simulink model "MJAUV_Maneuverability_model_V2"  (R2022b)
settings: Solver=ode4  StartTime=0.0  StopTime=50  FixedStep=0.0001  RelTol=1e-3  EnableMultiTasking=on
libraries: sharedutil x64, matrix_library x35
(part 2 of 5)

== system MJAUV_Maneuverability_model_V2/MJ-AUV Model & PropulsionSystem/Dynamics and Kinematics/6 DOF transformation/E1(e) ==
  note: qo
  note: q1,q2,q3
  e : Inport
  Gain : Gain  Gain=2  SaturateOnIntegerOverflow=on  OutDataTypeStr=Inherit: Same as input  ParamDataTypeStr=Inherit: Same as input
  "Gain " : Gain  Gain=2  SaturateOnIntegerOverflow=on  OutDataTypeStr=Inherit: Same as input  ParamDataTypeStr=Inherit: Same as input
  I (3x3) : Constant  Value=eye(3)
  Matrix Multiply : Product  Multiplication=Matrix(*)
  Product : Product  SaturateOnIntegerOverflow=on  OutDataTypeStr=Inherit: Same as first input
  Selector : Selector  InputPortWidth=4  IndexOptions=Index vector (dialog)  Indices=[1]  OutputSizes=1
  Selector1 : Selector  InputPortWidth=4  IndexOptions=Index vector (dialog)  Indices=[2 3 4]  OutputSizes=1
  Skew Symmetrical Operator : Subsystem
  Sum : Sum  Inputs=+++  SaturateOnIntegerOverflow=on
  E1 : Outport  VectorParamsAs1DForOutWhenUnconnected=off
  wires:
  Sum/1 -> E1/1
  Gain/1 -> Sum/3
  Product/1 -> Sum/2
  I (3x3)/1 -> Sum/1
  "Gain "/1 -> Product/1
  Matrix Multiply/1 -> Gain/1
  Skew Symmetrical Operator/1(S(V)) -> Product/2, Matrix Multiply/2, Matrix Multiply/1
  Selector1/1 -> Skew Symmetrical Operator/1(v)  "eps"
  Selector/1 -> "Gain "/1  "eta"
  e/1 -> Selector1/1, Selector/1

== system MJAUV_Maneuverability_model_V2/MJ-AUV Model & PropulsionSystem/Dynamics and Kinematics/6 DOF transformation/E2(e) ==
  note: 如果将串联维度参数设置为 1，且输入是二维矩阵，模块将执行垂直矩阵串联，并将输入矩阵上下堆叠以创建输出矩阵。
  note: q0
  note: q=(q1,q2,q3)
  e : Inport
  Gain : Gain  Gain=0.5  SaturateOnIntegerOverflow=on  OutDataTypeStr=Inherit: Same as input  ParamDataTypeStr=Inherit: Same as input
  Gain1 : Gain  Gain=-1  SaturateOnIntegerOverflow=on  OutDataTypeStr=Inherit: Same as input  ParamDataTypeStr=Inherit: Same as input
  I (3x3) : Constant  Value=eye(3)
  Matrix Concatenation : Concatenate  Mode=Multidimensional array
  Product : Product  SaturateOnIntegerOverflow=on  OutDataTypeStr=Inherit: Same as first input
  Selector : Selector  InputPortWidth=4  IndexOptions=Index vector (dialog)  Indices=[1]  OutputSizes=1
  Selector1 : Selector  InputPortWidth=4  IndexOptions=Index vector (dialog)  Indices=[2 3 4]  OutputSizes=1
  Skew Symmetrical Operator : Subsystem
  Sum : Sum  SaturateOnIntegerOverflow=on
  Transpose : Math  Operator=transpose  SignedPower=on
  E2 : Outport  VectorParamsAs1DForOutWhenUnconnected=off
  wires:
  Gain/1 -> E2/1
  Matrix Concatenation/1 -> Gain/1
  Sum/1 -> Matrix Concatenation/2
  Gain1/1 -> Matrix Concatenation/1  "-eps^T"
  Transpose/1 -> Gain1/1
  Skew Symmetrical Operator/1(S(V)) -> Sum/2  "S(eps)"
  Product/1 -> Sum/1  "eta*I"
  I (3x3)/1 -> Product/1
  e/1 -> Selector/1, Selector1/1
  Selector/1 -> Product/2  "eta"
  Selector1/1 -> Transpose/1, Skew Symmetrical Operator/1(v)  "eps"

== system MJAUV_Maneuverability_model_V2/MJ-AUV Model & PropulsionSystem/Dynamics and Kinematics/Quaternion normalisation/norm 1x4 vector ==
  Inport : Inport
  Plus : Sum  Inputs=++++
  Selector : Selector  InputPortWidth=4  IndexOptions=Index vector (dialog)  Indices=[1]  OutputSizes=1
  Selector1 : Selector  InputPortWidth=4  IndexOptions=Index vector (dialog)  Indices=[2]  OutputSizes=1
  Selector2 : Selector  InputPortWidth=4  IndexOptions=Index vector (dialog)  Indices=[3]  OutputSizes=1
  Selector3 : Selector  InputPortWidth=4  IndexOptions=Index vector (dialog)  Indices=[4]  OutputSizes=1
  Sqrt : Sqrt
  Square{,1..3} (4 alike) : Math  Operator=square  SignedPower=on
  norm : Outport  VectorParamsAs1DForOutWhenUnconnected=off
  wires:
  Selector/1 -> Square/1
  Selector1/1 -> Square1/1
  Sqrt/1 -> norm/1
  Selector2/1 -> Square2/1
  Plus/1 -> Sqrt/1
  Selector3/1 -> Square3/1
  Square3/1 -> Plus/4
  Inport/1 -> Selector1/1, Selector/1, Selector2/1, Selector3/1
  Square/1 -> Plus/1
  Square1/1 -> Plus/2
  Square2/1 -> Plus/3

== system MJAUV_Maneuverability_model_V2/MJ-AUV Model & PropulsionSystem/Dynamics and Kinematics/Subsystem1/H_BS ==
  R_BS : Inport
  Constant1 : Constant  Value=r_B
  Gain : Gain  Gain=-1
  Matrix Concatenation : Concatenate  Mode=Multidimensional array
  Matrix Concatenation1 : Concatenate  Mode=Multidimensional array
  Matrix Concatenation2 : Concatenate  Mode=Multidimensional array  ConcatenateDimension=2
  Matrix Multiply3 : Product  Multiplication=Matrix(*)
  "Skew Symmetrical Operator " : Subsystem
  Zero matrix (3 x 3) : Constant  Value=zeros(3,3)
  H_BS : Outport
  wires:
  Constant1/1 -> "Skew Symmetrical Operator "/1(v)
  "Skew Symmetrical Operator "/1(S(V)) -> Matrix Multiply3/2
  Gain/1 -> Matrix Concatenation/2  "R(1,2)"
  R_BS/1 -> Matrix Concatenation1/2, Matrix Concatenation/1, Matrix Multiply3/1
  Matrix Concatenation/1 -> Matrix Concatenation2/1
  Matrix Concatenation1/1 -> Matrix Concatenation2/2
  Matrix Multiply3/1 -> Gain/1
  Zero matrix (3 x 3)/1 -> Matrix Concatenation1/1  "R(2,1)"
  Matrix Concatenation2/1 -> H_BS/1

== system MJAUV_Maneuverability_model_V2/MJ-AUV Model & PropulsionSystem/Dynamics and Kinematics/Subsystem1/{B}->{S} Transformation ==
  v : Inport
  Constant : Constant  Value=0
  Constant1 : Constant
  Create 3x3 Matrix : sharedutil/Create 3x3 Matrix  aMode=aMode
  Gain : Gain  Gain=-1  SaturateOnIntegerOverflow=on  OutDataTypeStr=Inherit: Same as input  ParamDataTypeStr=Inherit: Same as input
  Trigonometric Function : Trigonometry  Operator=sincos
  R(v) : Outport  VectorParamsAs1DForOutWhenUnconnected=off
  wires:
  v/1 -> Trigonometric Function/1
  Create 3x3 Matrix/1 -> R(v)/1
  Constant/1 -> Create 3x3 Matrix/8, Create 3x3 Matrix/7, Create 3x3 Matrix/6, Create 3x3 Matrix/3
  Constant1/1 -> Create 3x3 Matrix/9
  Trigonometric Function/2 -> Create 3x3 Matrix/5, Create 3x3 Matrix/1
  Trigonometric Function/1 -> Gain/1, Create 3x3 Matrix/2
  Gain/1 -> Create 3x3 Matrix/4  "-v(1)"

== system MJAUV_Maneuverability_model_V2/MJ-AUV Model & PropulsionSystem/Dynamics and Kinematics/Subsystem2/H_ST ==
  R_ST : Inport
  Constant1 : Constant  Value=r_S
  Gain : Gain  Gain=-1
  Matrix Concatenation : Concatenate  Mode=Multidimensional array
  Matrix Concatenation1 : Concatenate  Mode=Multidimensional array
  Matrix Concatenation2 : Concatenate  Mode=Multidimensional array  ConcatenateDimension=2
  Matrix Multiply3 : Product  Multiplication=Matrix(*)
  "Skew Symmetrical Operator " : Subsystem
  Zero matrix (3 x 3) : Constant  Value=zeros(3,3)
  H_ST : Outport
  wires:
  Constant1/1 -> "Skew Symmetrical Operator "/1(v)
  "Skew Symmetrical Operator "/1(S(V)) -> Matrix Multiply3/2
  Gain/1 -> Matrix Concatenation/2  "R(1,2)"
  R_ST/1 -> Matrix Concatenation1/2, Matrix Concatenation/1, Matrix Multiply3/1
  Matrix Concatenation/1 -> Matrix Concatenation2/1
  Matrix Concatenation1/1 -> Matrix Concatenation2/2
  Matrix Multiply3/1 -> Gain/1
  Zero matrix (3 x 3)/1 -> Matrix Concatenation1/1  "R(2,1)"
  Matrix Concatenation2/1 -> H_ST/1

== system MJAUV_Maneuverability_model_V2/MJ-AUV Model & PropulsionSystem/Dynamics and Kinematics/Subsystem2/{S}->{T} Transformation ==
  v : Inport
  Constant : Constant  Value=0
  Constant1 : Constant
  Create 3x3 Matrix : sharedutil/Create 3x3 Matrix  aMode=aMode
  Gain : Gain  Gain=-1  SaturateOnIntegerOverflow=on  OutDataTypeStr=Inherit: Same as input  ParamDataTypeStr=Inherit: Same as input
  Trigonometric Function : Trigonometry  Operator=sincos
  R(v) : Outport  VectorParamsAs1DForOutWhenUnconnected=off
  wires:
  v/1 -> Trigonometric Function/1
  Create 3x3 Matrix/1 -> R(v)/1
  Constant/1 -> Create 3x3 Matrix/8, Create 3x3 Matrix/7, Create 3x3 Matrix/6, Create 3x3 Matrix/3
  Constant1/1 -> Create 3x3 Matrix/9
  Trigonometric Function/2 -> Create 3x3 Matrix/5, Create 3x3 Matrix/1
  Trigonometric Function/1 -> Gain/1, Create 3x3 Matrix/2
  Gain/1 -> Create 3x3 Matrix/4  "-v(1)"

== system MJAUV_Maneuverability_model_V2/MJ-AUV Model & PropulsionSystem/Dynamics and Kinematics/Subsystem3/H_TF ==
  R_TF : Inport
  Constant1 : Constant  Value=r_F
  Gain : Gain  Gain=-1
  Matrix Concatenation : Concatenate  Mode=Multidimensional array
  Matrix Concatenation1 : Concatenate  Mode=Multidimensional array
  Matrix Concatenation2 : Concatenate  Mode=Multidimensional array  ConcatenateDimension=2
  Matrix Multiply3 : Product  Multiplication=Matrix(*)
  "Skew Symmetrical Operator " : Subsystem
  Zero matrix (3 x 3) : Constant  Value=zeros(3,3)
  H_TF : Outport
  wires:
  Matrix Concatenation2/1 -> H_TF/1
  Zero matrix (3 x 3)/1 -> Matrix Concatenation1/1  "R(2,1)"
  Matrix Multiply3/1 -> Gain/1
  Matrix Concatenation1/1 -> Matrix Concatenation2/2
  Matrix Concatenation/1 -> Matrix Concatenation2/1
  R_TF/1 -> Matrix Multiply3/1, Matrix Concatenation/1, Matrix Concatenation1/2
  Gain/1 -> Matrix Concatenation/2  "R(1,2)"
  "Skew Symmetrical Operator "/1(S(V)) -> Matrix Multiply3/2
  Constant1/1 -> "Skew Symmetrical Operator "/1(v)

== system MJAUV_Maneuverability_model_V2/MJ-AUV Model & PropulsionSystem/Dynamics and Kinematics/Subsystem3/{T}->{F} Transformation ==
  v : Inport
  Constant : Constant  Value=0
  Constant1 : Constant
  Create 3x3 Matrix : sharedutil/Create 3x3 Matrix  aMode=aMode
  Gain : Gain  Gain=-1  SaturateOnIntegerOverflow=on  OutDataTypeStr=Inherit: Same as input  ParamDataTypeStr=Inherit: Same as input
  Trigonometric Function : Trigonometry  Operator=sincos
  R(v) : Outport  VectorParamsAs1DForOutWhenUnconnected=off
  wires:
  Gain/1 -> Create 3x3 Matrix/4  "-v(1)"
  Trigonometric Function/1 -> Create 3x3 Matrix/2, Gain/1
  Trigonometric Function/2 -> Create 3x3 Matrix/1, Create 3x3 Matrix/5
  Constant1/1 -> Create 3x3 Matrix/9
  Constant/1 -> Create 3x3 Matrix/3, Create 3x3 Matrix/6, Create 3x3 Matrix/7, Create 3x3 Matrix/8
  Create 3x3 Matrix/1 -> R(v)/1
  v/1 -> Trigonometric Function/1

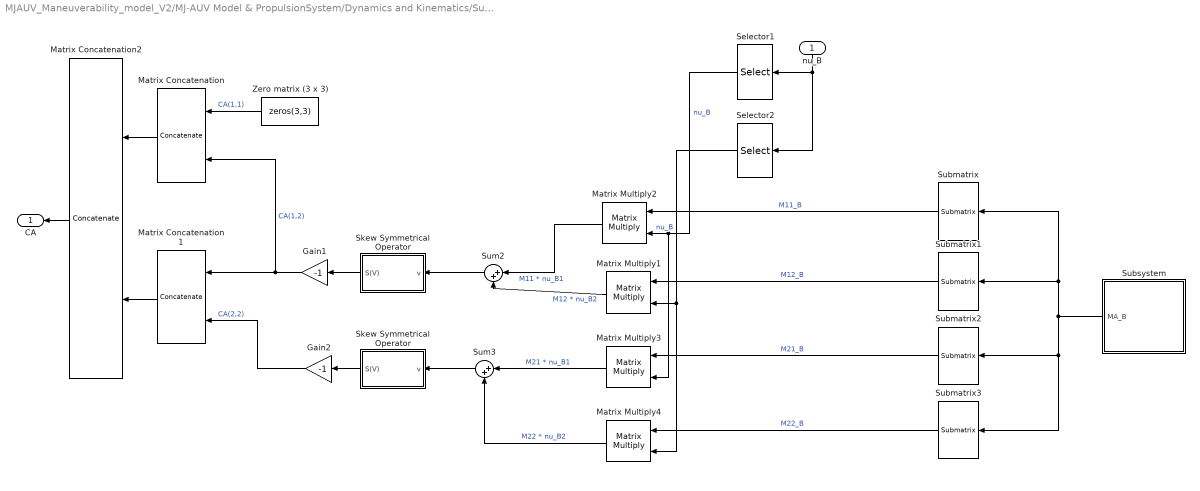
== system MJAUV_Maneuverability_model_V2/MJ-AUV Model & PropulsionSystem/Dynamics and Kinematics/Subsystem4/Added Mass Coriolis and centripetal matrix ==
  nu_B : Inport
  Gain1 : Gain  Gain=-1  SaturateOnIntegerOverflow=on  OutDataTypeStr=Inherit: Same as input  ParamDataTypeStr=Inherit: Same as input
  Gain2 : Gain  Gain=-1  SaturateOnIntegerOverflow=on  OutDataTypeStr=Inherit: Same as input  ParamDataTypeStr=Inherit: Same as input
  Matrix Concatenation : Concatenate  Mode=Multidimensional array
  Matrix Concatenation1 : Concatenate  Mode=Multidimensional array
  Matrix Concatenation2 : Concatenate  Mode=Multidimensional array  ConcatenateDimension=2
  Matrix Multiply{1..4} (4 alike) : Product  Multiplication=Matrix(*)
  Selector1 : Selector  InputPortWidth=6  IndexOptions=Index vector (dialog)  Indices=[1 2 3]  OutputSizes=1
  Selector2 : Selector  InputPortWidth=6  IndexOptions=Index vector (dialog)  Indices=[4 5 6]  OutputSizes=1
  Skew Symmetrical Operator : Subsystem
  "Skew Symmetrical Operator " : Subsystem
  Submatrix : matrix_library/Submatrix  RowSpan=Range of rows  RowStartMode=Index  RowStartIndex=1  RowEndMode=Index  RowEndIndex=3  ColSpan=Range of columns  ColStartMode=Index  ColStartIndex=1  ColEndMode=Index  ColEndIndex=3
  Submatrix1 : matrix_library/Submatrix  RowSpan=Range of rows  RowStartMode=Index  RowStartIndex=1  RowEndMode=Index  RowEndIndex=3  ColSpan=Range of columns  ColStartMode=Index  ColStartIndex=4  ColEndMode=Index  ColEndIndex=6
  Submatrix2 : matrix_library/Submatrix  RowSpan=Range of rows  RowStartMode=Index  RowStartIndex=4  RowEndMode=Index  RowEndIndex=6  ColSpan=Range of columns  ColStartMode=Index  ColStartIndex=1  ColEndMode=Index  ColEndIndex=3
  Submatrix3 : matrix_library/Submatrix  RowSpan=Range of rows  RowStartMode=Index  RowStartIndex=4  RowEndMode=Index  RowEndIndex=6  ColSpan=Range of columns  ColStartMode=Index  ColStartIndex=4  ColEndMode=Index  ColEndIndex=6
  Subsystem : Subsystem
  Sum2 : Sum  Inputs=|++  SaturateOnIntegerOverflow=on
  Sum3 : Sum  Inputs=|++  SaturateOnIntegerOverflow=on
  Zero matrix (3 x 3) : Constant  Value=zeros(3,3)
  CA : Outport  VectorParamsAs1DForOutWhenUnconnected=off
  wires:
  Submatrix3/1 -> Matrix Multiply4/1  "M22_B"
  Submatrix2/1 -> Matrix Multiply3/1  "M21_B"
  Submatrix1/1 -> Matrix Multiply1/1  "M12_B"
  Submatrix/1 -> Matrix Multiply2/1  "M11_B"
  Matrix Concatenation2/1 -> CA/1
  nu_B/1 -> Selector2/1, Selector1/1
  Gain2/1 -> Matrix Concatenation1/2  "CA(2,2)"
  Gain1/1 -> Matrix Concatenation/2, Matrix Concatenation1/1  "CA(1,2)"
  Skew Symmetrical Operator/1(S(V)) -> Gain2/1
  "Skew Symmetrical Operator "/1(S(V)) -> Gain1/1
  Sum3/1 -> Skew Symmetrical Operator/1(v)
  Sum2/1 -> "Skew Symmetrical Operator "/1(v)
  Selector2/1 -> Matrix Multiply4/2, Matrix Multiply1/2  "nu_B"
  Matrix Multiply4/1 -> Sum3/2  "M22 * nu_B2"
  Selector1/1 -> Matrix Multiply3/2, Matrix Multiply2/2  "nu_B"
  Matrix Multiply3/1 -> Sum3/1  "M21 * nu_B1"
  Matrix Multiply1/1 -> Sum2/2  "M12 * nu_B2"
  Matrix Multiply2/1 -> Sum2/1  "M11 * nu_B1"
  Matrix Concatenation1/1 -> Matrix Concatenation2/2
  Matrix Concatenation/1 -> Matrix Concatenation2/1
  Zero matrix (3 x 3)/1 -> Matrix Concatenation/1  "CA(1,1)"
  Subsystem/1(MA_B) -> Submatrix/1, Submatrix1/1, Submatrix3/1, Submatrix2/1

== system MJAUV_Maneuverability_model_V2/MJ-AUV Model & PropulsionSystem/Dynamics and Kinematics/Subsystem4/Damping forces ==
  nu_B : Inport
  Abs : Abs
  Create Diagonal Matrix : matrix_library/Create Diagonal Matrix
  Gain : Gain  Gain=-1
  Linear Damping Matrix : Constant  Value=DL
  Matrix Multiply : Product  Multiplication=Matrix(*)
  Product : Product  SaturateOnIntegerOverflow=on  OutDataTypeStr=Inherit: Same as first input
  Quadratic Damping Vector : Constant  Value=dQ_B
  Reshape1 : Reshape  OutputDimensionality=Column vector (2-D)
  Reshape2 : Reshape  OutputDimensionality=Column vector (2-D)  OutputDimensions=[6,6]
  Sum1 : Sum  Inputs=|++  SaturateOnIntegerOverflow=on
  D * nu_B : Outport  VectorParamsAs1DForOutWhenUnconnected=off
  wires:
  Gain/1 -> Matrix Multiply/1
  Sum1/1 -> Gain/1  "D"
  Matrix Multiply/1 -> D * nu_B/1
  Quadratic Damping Vector/1 -> Reshape2/1  "dQ"
  Abs/1 -> Product/2  "abs(nu_B)"
  Product/1 -> Create Diagonal Matrix/1
  Create Diagonal Matrix/1 -> Sum1/2
  Linear Damping Matrix/1 -> Sum1/1
  nu_B/1 -> Reshape1/1
  Reshape1/1 -> Abs/1, Matrix Multiply/2
  Reshape2/1 -> Product/1

== system MJAUV_Maneuverability_model_V2/MJ-AUV Model & PropulsionSystem/Dynamics and Kinematics/Subsystem4/Restoring forces ==
  eta_E : Inport
  3x3 Cross Product : sharedutil/3x3 Cross Product  aMode=aMode
  3x3 Cross Product1 : sharedutil/3x3 Cross Product  aMode=aMode
  E1(e) : Subsystem
  Gain : Gain  Gain=-1  SaturateOnIntegerOverflow=on  OutDataTypeStr=Inherit: Same as input  ParamDataTypeStr=Inherit: Same as input
  Matrix Multiply : Product  Multiplication=Matrix(*)
  Matrix Multiply1 : Product  Multiplication=Matrix(*)
  Mux : Mux  Inputs=2
  Selector : Selector  InputPortWidth=7  IndexOptions=Index vector (dialog)  Indices=[4 5 6 7]  OutputSizes=1
  Sum1 : Sum  Inputs=|++  SaturateOnIntegerOverflow=on
  Sum2 : Sum  Inputs=|++  SaturateOnIntegerOverflow=on
  Transpose : Math  Operator=transpose  SignedPower=on
  fBB_E : Constant  Value=[0;0;-B_B]
  fGB_E : Constant  Value=[0;0;W_B]
  rB_B : Constant  Value=rB_B
  rG_B : Constant  Value=rG_B
  g(eta_E)_B : Outport  VectorParamsAs1DForOutWhenUnconnected=off
  wires:
  eta_E/1 -> Selector/1  "E1(e)"
  Selector/1 -> E1(e)/1(e)  "e"
  Gain/1 -> g(eta_E)_B/1
  Mux/1 -> Gain/1
  Sum2/1 -> Mux/2
  rB_B/1 -> 3x3 Cross Product1/1
  3x3 Cross Product1/1 -> Sum2/2  "rG_B x fG_B"
  3x3 Cross Product/1 -> Sum2/1  "rG_B x fG_B"
  Sum1/1 -> Mux/1  "fG_B + fB_B"
  rG_B/1 -> 3x3 Cross Product/1
  Matrix Multiply1/1 -> 3x3 Cross Product1/2, Sum1/2  "fB_B"
  Matrix Multiply/1 -> 3x3 Cross Product/2, Sum1/1  "fG_B"
  fBB_E/1 -> Matrix Multiply1/2
  fGB_E/1 -> Matrix Multiply/2
  Transpose/1 -> Matrix Multiply1/1, Matrix Multiply/1  "E1(e)^T"
  E1(e)/1(E1) -> Transpose/1  "E1(e)"

== system MJAUV_Maneuverability_model_V2/MJ-AUV Model & PropulsionSystem/Dynamics and Kinematics/Subsystem4/Rigid-body Coriolis and centripetal matrix ==
  nu_B : Inport
  Gain : Gain  Gain=mB  SaturateOnIntegerOverflow=on  OutDataTypeStr=Inherit: Same as input  ParamDataTypeStr=Inherit: Same as input
  Gain1 : Gain  Gain=-mB  SaturateOnIntegerOverflow=on  OutDataTypeStr=Inherit: Same as input  ParamDataTypeStr=Inherit: Same as input
  Gain2 : Gain  Gain=-1  SaturateOnIntegerOverflow=on  OutDataTypeStr=Inherit: Same as input  ParamDataTypeStr=Inherit: Same as input
  Matrix Concatenation : Concatenate  Mode=Multidimensional array
  Matrix Concatenation1 : Concatenate  Mode=Multidimensional array
  Matrix Concatenation2 : Concatenate  Mode=Multidimensional array  ConcatenateDimension=2
  Matrix Multiply : Product  Multiplication=Matrix(*)
  Matrix Multiply1 : Product  Multiplication=Matrix(*)
  Matrix Multiply2 : Product  Multiplication=Matrix(*)
  Selector : Selector  InputPortWidth=6  IndexOptions=Index vector (dialog)  Indices=[4 5 6]  OutputSizes=1
  Selector1 : Selector  InputPortWidth=6  IndexOptions=Index vector (dialog)  Indices=[1 2 3]  OutputSizes=1
  "Skew Symmetrical Operator " : Subsystem
  Skew Symmetrical Operator : Subsystem
  "Skew Symmetrical Operator " : Subsystem
  "Skew Symmetrical Operator  " : Subsystem
  Subsystem : Subsystem
  Sum1 : Sum  Inputs=|++  SaturateOnIntegerOverflow=on
  Sum2 : Sum  Inputs=|-+  SaturateOnIntegerOverflow=on
  Zero matrix (3 x 3) : Constant  Value=zeros(3,3)
  rG_B : Constant  Value=rG_B
  CRB : Outport  VectorParamsAs1DForOutWhenUnconnected=off
  wires:
  "Skew Symmetrical Operator  "/1(S(V)) -> Matrix Multiply1/2, Matrix Multiply/1  "S(rG_B)"
  Matrix Multiply1/1 -> Sum1/2  "S(nu2_B) * S(rG_B)"
  Sum1/1 -> Gain1/1
  "Skew Symmetrical Operator "/1(S(V)) -> Matrix Multiply1/1, Matrix Multiply/2  "S(nu2_B)"
  Matrix Concatenation/1 -> Matrix Concatenation2/1
  Subsystem/1(Ib_B) -> Matrix Multiply2/1
  Matrix Multiply/1 -> Sum2/2  "S(rG_B) * S(nu2_B)"
  Selector/1 -> Matrix Multiply2/2, "Skew Symmetrical Operator "/1(v)  "nu2_B"
  Matrix Concatenation1/1 -> Matrix Concatenation2/2
  Sum2/1 -> Gain/1
  Matrix Multiply2/1 -> "Skew Symmetrical Operator "/1(v)  "IO * nu2_B"
  Zero matrix (3 x 3)/1 -> Matrix Concatenation/1  "CRB(1,1)"
  Gain1/1 -> Matrix Concatenation1/1  "CRB(1,2)"
  Skew Symmetrical Operator/1(S(V)) -> Sum1/1, Sum2/1  "S(nu1_B)"
  Matrix Concatenation2/1 -> CRB/1
  nu_B/1 -> Selector1/1, Selector/1
  Selector1/1 -> Skew Symmetrical Operator/1(v)  "nu1_B"
  "Skew Symmetrical Operator "/1(S(V)) -> Gain2/1  "S(IO * nu2_B)"
  rG_B/1 -> "Skew Symmetrical Operator  "/1(v), Subsystem/1(rG_B)  "rG_B"
  Gain/1 -> Matrix Concatenation/2  "CRB(2,1)"
  Gain2/1 -> Matrix Concatenation1/2  "CRB(2,2)"

== system MJAUV_Maneuverability_model_V2/MJ-AUV Model & PropulsionSystem/Dynamics and Kinematics/Subsystem5/K ==
  R_FT : Inport
  Constant1 : Constant  Value=r_T
  Gain : Gain  Gain=-1
  Matrix Concatenation : Concatenate  Mode=Multidimensional array
  Matrix Concatenation1 : Concatenate  Mode=Multidimensional array
  Matrix Concatenation2 : Concatenate  Mode=Multidimensional array  ConcatenateDimension=2
  Matrix Multiply3 : Product  Multiplication=Matrix(*)
  "Skew Symmetrical Operator " : Subsystem
  Zero matrix (3 x 3) : Constant  Value=zeros(3,3)
  K_FT : Outport
  wires:
  Matrix Concatenation2/1 -> K_FT/1
  Zero matrix (3 x 3)/1 -> Matrix Concatenation1/1  "R(2,1)"
  Matrix Multiply3/1 -> Gain/1
  Matrix Concatenation1/1 -> Matrix Concatenation2/2
  Matrix Concatenation/1 -> Matrix Concatenation2/1
  R_FT/1 -> Matrix Multiply3/1, Matrix Concatenation/1, Matrix Concatenation1/2
  Gain/1 -> Matrix Concatenation/2  "R(1,2)"
  "Skew Symmetrical Operator "/1(S(V)) -> Matrix Multiply3/2
  Constant1/1 -> "Skew Symmetrical Operator "/1(v)

== system MJAUV_Maneuverability_model_V2/MJ-AUV Model & PropulsionSystem/Dynamics and Kinematics/Subsystem5/K_B ==
  R_SB : Inport
  Constant1 : Constant  Value=r_B
  Gain : Gain  Gain=-1
  Matrix Concatenation : Concatenate  Mode=Multidimensional array
  Matrix Concatenation1 : Concatenate  Mode=Multidimensional array
  Matrix Concatenation2 : Concatenate  Mode=Multidimensional array  ConcatenateDimension=2
  Matrix Multiply3 : Product  Multiplication=Matrix(*)
  "Skew Symmetrical Operator " : Subsystem
  Zero matrix (3 x 3) : Constant  Value=zeros(3,3)
  K_SB : Outport
  wires:
  Constant1/1 -> "Skew Symmetrical Operator "/1(v)
  "Skew Symmetrical Operator "/1(S(V)) -> Matrix Multiply3/2
  Gain/1 -> Matrix Concatenation1/1  "R(1,2)"
  R_SB/1 -> Matrix Concatenation1/2, Matrix Concatenation/1, Matrix Multiply3/1
  Matrix Concatenation/1 -> Matrix Concatenation2/1
  Matrix Concatenation1/1 -> Matrix Concatenation2/2
  Matrix Multiply3/1 -> Gain/1
  Zero matrix (3 x 3)/1 -> Matrix Concatenation/2  "R(2,1)"
  Matrix Concatenation2/1 -> K_SB/1

== system MJAUV_Maneuverability_model_V2/MJ-AUV Model & PropulsionSystem/Dynamics and Kinematics/Subsystem5/K_T ==
  R_TS : Inport
  Constant1 : Constant  Value=r_S
  Gain : Gain  Gain=-1
  Matrix Concatenation : Concatenate  Mode=Multidimensional array
  Matrix Concatenation1 : Concatenate  Mode=Multidimensional array
  Matrix Concatenation2 : Concatenate  Mode=Multidimensional array  ConcatenateDimension=2
  Matrix Multiply3 : Product  Multiplication=Matrix(*)
  "Skew Symmetrical Operator " : Subsystem
  Zero matrix (3 x 3) : Constant  Value=zeros(3,3)
  K_TS : Outport
  wires:
  Constant1/1 -> "Skew Symmetrical Operator "/1(v)
  "Skew Symmetrical Operator "/1(S(V)) -> Matrix Multiply3/2
  Gain/1 -> Matrix Concatenation1/1  "R(1,2)"
  R_TS/1 -> Matrix Concatenation1/2, Matrix Concatenation/1, Matrix Multiply3/1
  Matrix Concatenation/1 -> Matrix Concatenation2/1
  Matrix Concatenation1/1 -> Matrix Concatenation2/2
  Matrix Multiply3/1 -> Gain/1
  Zero matrix (3 x 3)/1 -> Matrix Concatenation/2  "R(2,1)"
  Matrix Concatenation2/1 -> K_TS/1

== system MJAUV_Maneuverability_model_V2/MJ-AUV Model & PropulsionSystem/Dynamics and Kinematics/Subsystem5/{B}->{S} Transformation ==
  v : Inport
  Constant : Constant  Value=0
  Constant1 : Constant
  Create 3x3 Matrix : sharedutil/Create 3x3 Matrix  aMode=aMode
  Gain : Gain  Gain=-1  SaturateOnIntegerOverflow=on  OutDataTypeStr=Inherit: Same as input  ParamDataTypeStr=Inherit: Same as input
  Trigonometric Function : Trigonometry  Operator=sincos
  R(v) : Outport  VectorParamsAs1DForOutWhenUnconnected=off
  wires:
  v/1 -> Trigonometric Function/1
  Create 3x3 Matrix/1 -> R(v)/1
  Constant/1 -> Create 3x3 Matrix/8, Create 3x3 Matrix/7, Create 3x3 Matrix/6, Create 3x3 Matrix/3
  Constant1/1 -> Create 3x3 Matrix/9
  Trigonometric Function/2 -> Create 3x3 Matrix/5, Create 3x3 Matrix/1
  Trigonometric Function/1 -> Gain/1, Create 3x3 Matrix/2
  Gain/1 -> Create 3x3 Matrix/4  "-v(1)"

== system MJAUV_Maneuverability_model_V2/MJ-AUV Model & PropulsionSystem/Dynamics and Kinematics/Subsystem5/{S}->{T} Transformation ==
  v : Inport
  Constant : Constant  Value=0
  Constant1 : Constant
  Create 3x3 Matrix : sharedutil/Create 3x3 Matrix  aMode=aMode
  Gain : Gain  Gain=-1  SaturateOnIntegerOverflow=on  OutDataTypeStr=Inherit: Same as input  ParamDataTypeStr=Inherit: Same as input
  Trigonometric Function : Trigonometry  Operator=sincos
  R(v) : Outport  VectorParamsAs1DForOutWhenUnconnected=off
  wires:
  v/1 -> Trigonometric Function/1
  Create 3x3 Matrix/1 -> R(v)/1
  Constant/1 -> Create 3x3 Matrix/8, Create 3x3 Matrix/7, Create 3x3 Matrix/6, Create 3x3 Matrix/3
  Constant1/1 -> Create 3x3 Matrix/9
  Trigonometric Function/2 -> Create 3x3 Matrix/5, Create 3x3 Matrix/1
  Trigonometric Function/1 -> Gain/1, Create 3x3 Matrix/2
  Gain/1 -> Create 3x3 Matrix/4  "-v(1)"

== system MJAUV_Maneuverability_model_V2/MJ-AUV Model & PropulsionSystem/Dynamics and Kinematics/Subsystem5/{T}->{F} Transformation ==
  v : Inport
  Constant : Constant  Value=0
  Constant1 : Constant
  Create 3x3 Matrix : sharedutil/Create 3x3 Matrix  aMode=aMode
  Gain : Gain  Gain=-1  SaturateOnIntegerOverflow=on  OutDataTypeStr=Inherit: Same as input  ParamDataTypeStr=Inherit: Same as input
  Trigonometric Function : Trigonometry  Operator=sincos
  R(v) : Outport  VectorParamsAs1DForOutWhenUnconnected=off
  wires:
  Gain/1 -> Create 3x3 Matrix/4  "-v(1)"
  Trigonometric Function/1 -> Create 3x3 Matrix/2, Gain/1
  Trigonometric Function/2 -> Create 3x3 Matrix/1, Create 3x3 Matrix/5
  Constant1/1 -> Create 3x3 Matrix/9
  Constant/1 -> Create 3x3 Matrix/3, Create 3x3 Matrix/6, Create 3x3 Matrix/7, Create 3x3 Matrix/8
  Create 3x3 Matrix/1 -> R(v)/1
  v/1 -> Trigonometric Function/1

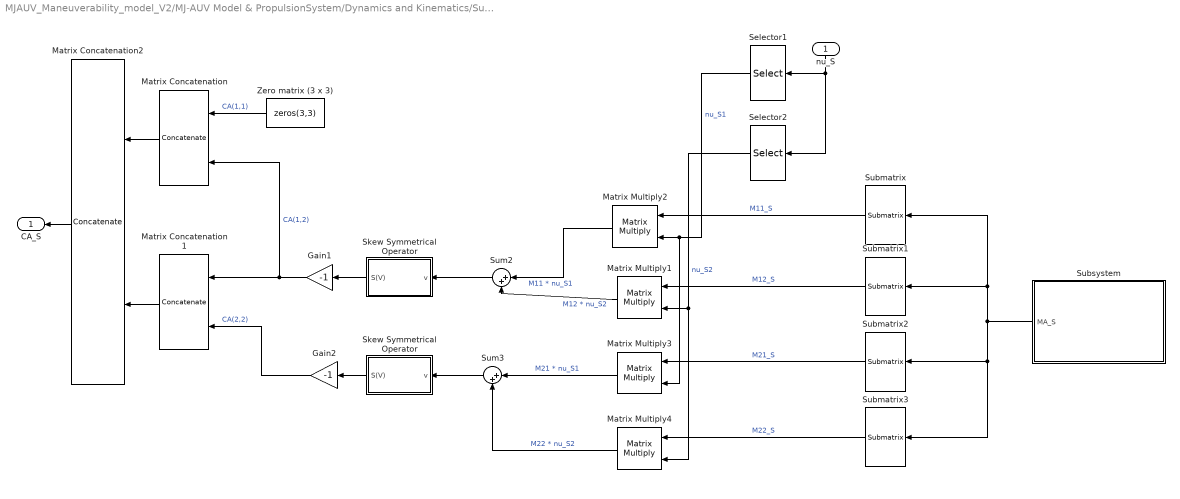
== system MJAUV_Maneuverability_model_V2/MJ-AUV Model & PropulsionSystem/Dynamics and Kinematics/Subsystem6/Added Mass Coriolis and centripetal matrix1 ==
  nu_S : Inport
  Gain1 : Gain  Gain=-1  SaturateOnIntegerOverflow=on  OutDataTypeStr=Inherit: Same as input  ParamDataTypeStr=Inherit: Same as input
  Gain2 : Gain  Gain=-1  SaturateOnIntegerOverflow=on  OutDataTypeStr=Inherit: Same as input  ParamDataTypeStr=Inherit: Same as input
  Matrix Concatenation : Concatenate  Mode=Multidimensional array
  Matrix Concatenation1 : Concatenate  Mode=Multidimensional array
  Matrix Concatenation2 : Concatenate  Mode=Multidimensional array  ConcatenateDimension=2
  Matrix Multiply{1..4} (4 alike) : Product  Multiplication=Matrix(*)
  Selector1 : Selector  InputPortWidth=6  IndexOptions=Index vector (dialog)  Indices=[1 2 3]  OutputSizes=1
  Selector2 : Selector  InputPortWidth=6  IndexOptions=Index vector (dialog)  Indices=[4 5 6]  OutputSizes=1
  Skew Symmetrical Operator : Subsystem
  "Skew Symmetrical Operator " : Subsystem
  Submatrix : matrix_library/Submatrix  RowSpan=Range of rows  RowStartMode=Index  RowStartIndex=1  RowEndMode=Index  RowEndIndex=3  ColSpan=Range of columns  ColStartMode=Index  ColStartIndex=1  ColEndMode=Index  ColEndIndex=3
  Submatrix1 : matrix_library/Submatrix  RowSpan=Range of rows  RowStartMode=Index  RowStartIndex=1  RowEndMode=Index  RowEndIndex=3  ColSpan=Range of columns  ColStartMode=Index  ColStartIndex=4  ColEndMode=Index  ColEndIndex=6
  Submatrix2 : matrix_library/Submatrix  RowSpan=Range of rows  RowStartMode=Index  RowStartIndex=4  RowEndMode=Index  RowEndIndex=6  ColSpan=Range of columns  ColStartMode=Index  ColStartIndex=1  ColEndMode=Index  ColEndIndex=3
  Submatrix3 : matrix_library/Submatrix  RowSpan=Range of rows  RowStartMode=Index  RowStartIndex=4  RowEndMode=Index  RowEndIndex=6  ColSpan=Range of columns  ColStartMode=Index  ColStartIndex=4  ColEndMode=Index  ColEndIndex=6
  Subsystem : Subsystem
  Sum2 : Sum  Inputs=|++  SaturateOnIntegerOverflow=on
  Sum3 : Sum  Inputs=|++  SaturateOnIntegerOverflow=on
  Zero matrix (3 x 3) : Constant  Value=zeros(3,3)
  CA_S : Outport  VectorParamsAs1DForOutWhenUnconnected=off
  wires:
  Zero matrix (3 x 3)/1 -> Matrix Concatenation/1  "CA(1,1)"
  Matrix Concatenation/1 -> Matrix Concatenation2/1
  Matrix Concatenation1/1 -> Matrix Concatenation2/2
  Matrix Multiply2/1 -> Sum2/1  "M11 * nu_S1"
  Matrix Multiply1/1 -> Sum2/2  "M12 * nu_S2"
  Matrix Multiply3/1 -> Sum3/1  "M21 * nu_S1"
  Selector1/1 -> Matrix Multiply2/2, Matrix Multiply3/2  "nu_S1"
  Matrix Multiply4/1 -> Sum3/2  "M22 * nu_S2"
  Selector2/1 -> Matrix Multiply1/2, Matrix Multiply4/2  "nu_S2"
  Sum2/1 -> "Skew Symmetrical Operator "/1(v)
  Sum3/1 -> Skew Symmetrical Operator/1(v)
  "Skew Symmetrical Operator "/1(S(V)) -> Gain1/1
  Skew Symmetrical Operator/1(S(V)) -> Gain2/1
  Gain1/1 -> Matrix Concatenation1/1, Matrix Concatenation/2  "CA(1,2)"
  Gain2/1 -> Matrix Concatenation1/2  "CA(2,2)"
  nu_S/1 -> Selector1/1, Selector2/1
  Matrix Concatenation2/1 -> CA_S/1
  Subsystem/1(MA_S) -> Submatrix/1, Submatrix1/1, Submatrix3/1, Submatrix2/1
  Submatrix3/1 -> Matrix Multiply4/1  "M22_S"
  Submatrix1/1 -> Matrix Multiply1/1  "M12_S"
  Submatrix2/1 -> Matrix Multiply3/1  "M21_S"
  Submatrix/1 -> Matrix Multiply2/1  "M11_S"

== system MJAUV_Maneuverability_model_V2/MJ-AUV Model & PropulsionSystem/Dynamics and Kinematics/Subsystem6/Damping forces1 ==
  nu_S : Inport
  Abs : Abs
  Create Diagonal Matrix : matrix_library/Create Diagonal Matrix
  Gain : Gain  Gain=-1
  Linear Damping Matrix : Constant  Value=DL
  Matrix Multiply : Product  Multiplication=Matrix(*)
  Product : Product  SaturateOnIntegerOverflow=on  OutDataTypeStr=Inherit: Same as first input
  Quadratic Damping Vector : Constant  Value=dQ_S
  Reshape1 : Reshape  OutputDimensionality=Column vector (2-D)
  Reshape2 : Reshape  OutputDimensionality=Column vector (2-D)  OutputDimensions=[6,6]
  Sum1 : Sum  Inputs=|++  SaturateOnIntegerOverflow=on
  D * nu_S : Outport  VectorParamsAs1DForOutWhenUnconnected=off
  wires:
  Reshape2/1 -> Product/1
  Reshape1/1 -> Matrix Multiply/2, Abs/1
  nu_S/1 -> Reshape1/1
  Linear Damping Matrix/1 -> Sum1/1
  Create Diagonal Matrix/1 -> Sum1/2
  Product/1 -> Create Diagonal Matrix/1
  Abs/1 -> Product/2  "abs(nu_S)"
  Quadratic Damping Vector/1 -> Reshape2/1  "dQ"
  Matrix Multiply/1 -> D * nu_S/1
  Sum1/1 -> Gain/1  "D"
  Gain/1 -> Matrix Multiply/1

== system MJAUV_Maneuverability_model_V2/MJ-AUV Model & PropulsionSystem/Dynamics and Kinematics/Subsystem6/Restoring forces1 ==
  eta_E : Inport
  rG_S : Inport  Port=2
  3x3 Cross Product : sharedutil/3x3 Cross Product  aMode=aMode
  3x3 Cross Product1 : sharedutil/3x3 Cross Product  aMode=aMode
  E1(e) : Subsystem
  Gain : Gain  Gain=-1  SaturateOnIntegerOverflow=on  OutDataTypeStr=Inherit: Same as input  ParamDataTypeStr=Inherit: Same as input
  Matrix Multiply : Product  Multiplication=Matrix(*)
  Matrix Multiply1 : Product  Multiplication=Matrix(*)
  Mux : Mux  Inputs=2
  Selector : Selector  InputPortWidth=7  IndexOptions=Index vector (dialog)  Indices=[4 5 6 7]  OutputSizes=1
  Sum1 : Sum  Inputs=|++  SaturateOnIntegerOverflow=on
  Sum2 : Sum  Inputs=|++  SaturateOnIntegerOverflow=on
  Transpose : Math  Operator=transpose  SignedPower=on
  fBS_E : Constant  Value=[0;0;-B_S]
  fGS_E : Constant  Value=[0;0;W_S]
  rB_S : Constant  Value=rB_S
  g(eta_E)_S : Outport  VectorParamsAs1DForOutWhenUnconnected=off
  wires:
  E1(e)/1(E1) -> Transpose/1  "E1(e)"
  Transpose/1 -> Matrix Multiply/1, Matrix Multiply1/1  "E1(e)^T"
  fGS_E/1 -> Matrix Multiply/2
  fBS_E/1 -> Matrix Multiply1/2
  Matrix Multiply/1 -> Sum1/1, 3x3 Cross Product/2  "fG_S"
  Matrix Multiply1/1 -> Sum1/2, 3x3 Cross Product1/2  "fB_S"
  rG_S/1 -> 3x3 Cross Product/1
  Sum1/1 -> Mux/1  "fG_S + fB_S"
  3x3 Cross Product/1 -> Sum2/1  "rG_S x fG_S"
  3x3 Cross Product1/1 -> Sum2/2  "rB_S x fG_S"
  rB_S/1 -> 3x3 Cross Product1/1
  Sum2/1 -> Mux/2
  Mux/1 -> Gain/1
  Gain/1 -> g(eta_E)_S/1
  Selector/1 -> E1(e)/1(e)  "e"
  eta_E/1 -> Selector/1  "E1(e)"

== system MJAUV_Maneuverability_model_V2/MJ-AUV Model & PropulsionSystem/Dynamics and Kinematics/Subsystem6/Rigid-body Coriolis and centripetal matrix1 ==
  nu_S : Inport
  rG_S : Inport  Port=2
  Gain : Gain  Gain=mS  SaturateOnIntegerOverflow=on  OutDataTypeStr=Inherit: Same as input  ParamDataTypeStr=Inherit: Same as input
  Gain1 : Gain  Gain=-mS  SaturateOnIntegerOverflow=on  OutDataTypeStr=Inherit: Same as input  ParamDataTypeStr=Inherit: Same as input
  Gain2 : Gain  Gain=-1  SaturateOnIntegerOverflow=on  OutDataTypeStr=Inherit: Same as input  ParamDataTypeStr=Inherit: Same as input
  Matrix Concatenation : Concatenate  Mode=Multidimensional array
  Matrix Concatenation1 : Concatenate  Mode=Multidimensional array
  Matrix Concatenation2 : Concatenate  Mode=Multidimensional array  ConcatenateDimension=2
  Matrix Multiply : Product  Multiplication=Matrix(*)
  Matrix Multiply1 : Product  Multiplication=Matrix(*)
  Matrix Multiply2 : Product  Multiplication=Matrix(*)
  Selector : Selector  InputPortWidth=6  IndexOptions=Index vector (dialog)  Indices=[4 5 6]  OutputSizes=1
  Selector1 : Selector  InputPortWidth=6  IndexOptions=Index vector (dialog)  Indices=[1 2 3]  OutputSizes=1
  "Skew Symmetrical Operator " : Subsystem
  Skew Symmetrical Operator : Subsystem
  "Skew Symmetrical Operator " : Subsystem
  "Skew Symmetrical Operator  " : Subsystem
  Subsystem : Subsystem
  Sum1 : Sum  Inputs=|++  SaturateOnIntegerOverflow=on
  Sum2 : Sum  Inputs=|-+  SaturateOnIntegerOverflow=on
  Zero matrix (3 x 3) : Constant  Value=zeros(3,3)
  CRB_S : Outport  VectorParamsAs1DForOutWhenUnconnected=off
  wires:
  Gain2/1 -> Matrix Concatenation1/2  "CRB(2,2)"
  Gain/1 -> Matrix Concatenation/2  "CRB(2,1)"
  "Skew Symmetrical Operator "/1(S(V)) -> Gain2/1  "S(IO * nu_S2)"
  Selector1/1 -> Skew Symmetrical Operator/1(v)  "nu_S1"
  nu_S/1 -> Selector/1, Selector1/1
  Matrix Concatenation2/1 -> CRB_S/1
  Skew Symmetrical Operator/1(S(V)) -> Sum2/1, Sum1/1  "S(nu_S1)"
  Gain1/1 -> Matrix Concatenation1/1  "CRB(1,2)"
  Zero matrix (3 x 3)/1 -> Matrix Concatenation/1  "CRB(1,1)"
  Matrix Multiply2/1 -> "Skew Symmetrical Operator "/1(v)  "IO * nu_S2"
  Sum2/1 -> Gain/1
  Matrix Concatenation1/1 -> Matrix Concatenation2/2
  Selector/1 -> "Skew Symmetrical Operator "/1(v), Matrix Multiply2/2  "nu_S2"
  Matrix Multiply/1 -> Sum2/2  "S(rG_S) * S(nu_S2)"
  Subsystem/1(Ib_S) -> Matrix Multiply2/1
  Matrix Concatenation/1 -> Matrix Concatenation2/1
  "Skew Symmetrical Operator "/1(S(V)) -> Matrix Multiply/2, Matrix Multiply1/1  "S(nu_S2)"
  Sum1/1 -> Gain1/1
  Matrix Multiply1/1 -> Sum1/2  "S(nu_S2) * S(rG_S)"
  "Skew Symmetrical Operator  "/1(S(V)) -> Matrix Multiply/1, Matrix Multiply1/2  "S(rG_S)"
  rG_S/1 -> "Skew Symmetrical Operator  "/1(v), Subsystem/1(rG_S)  "rG_S"

== system MJAUV_Maneuverability_model_V2/MJ-AUV Model & PropulsionSystem/Dynamics and Kinematics/Subsystem6/Subsystem1 ==
  eta_E_B : Inport
  Theta : Inport  Port=2
  Demux : Demux  Outputs=3
  Mux : Mux  Inputs=3
  Mux1 : Mux  Inputs=2
  Quaternion normalisation : Subsystem
  Quaternions to Euler Angles : Subsystem
  Scope : Scope  NumInputPorts=2
  Selector : Selector  InputPortWidth=7  IndexOptions=Index vector (dialog)  Indices=[4 5 6 7]  OutputSizes=1
  Selector1 : Selector  InputPortWidth=3  IndexOptions=Index vector (dialog)  Indices=[1]  OutputSizes=1
  Selector2 : Selector  InputPortWidth=7  IndexOptions=Index vector (dialog)  Indices=[1 2 3]  OutputSizes=1
  Subsystem : Subsystem
  Subsystem1 : Subsystem
  Sum : Sum  Inputs=|++
  eta_E_S : Outport
  wires:
  eta_E_B/1 -> Selector2/1, Selector/1
  Selector/1 -> Quaternions to Euler Angles/1(Quaternions)  "e"
  Demux/2 -> Mux/2
  Demux/3 -> Sum/1, Scope/2
  Quaternions to Euler Angles/1(Euler Angles) -> Demux/1
  Subsystem/1(Quaternions) -> Mux1/2
  Selector1/1 -> Sum/2  "Theta1"
  Selector2/1 -> Mux1/1  "e"
  Mux/1 -> Subsystem/1("Euler Angles ")
  Demux/1 -> Mux/1
  Mux1/1 -> Quaternion normalisation/1(eta_E)
  Sum/1 -> Subsystem1/1(In2)
  Quaternion normalisation/1(eta_E (norm)) -> eta_E_S/1
  Theta/1 -> Selector1/1
  Subsystem1/1(Out1) -> Scope/1, Mux/3

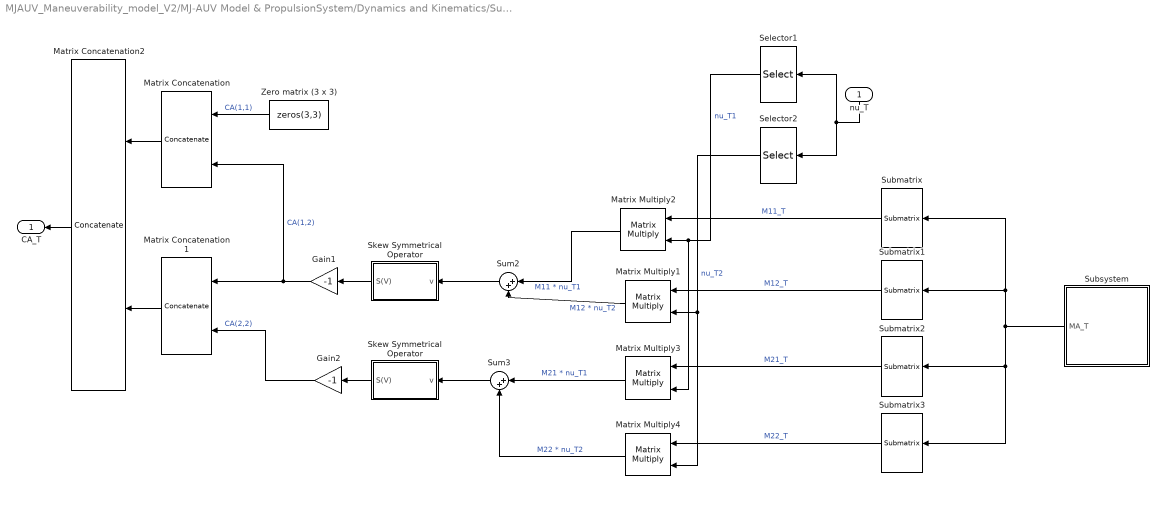
== system MJAUV_Maneuverability_model_V2/MJ-AUV Model & PropulsionSystem/Dynamics and Kinematics/Subsystem7/Added Mass Coriolis and centripetal matrix1 ==
  nu_T : Inport
  Gain1 : Gain  Gain=-1  SaturateOnIntegerOverflow=on  OutDataTypeStr=Inherit: Same as input  ParamDataTypeStr=Inherit: Same as input
  Gain2 : Gain  Gain=-1  SaturateOnIntegerOverflow=on  OutDataTypeStr=Inherit: Same as input  ParamDataTypeStr=Inherit: Same as input
  Matrix Concatenation : Concatenate  Mode=Multidimensional array
  Matrix Concatenation1 : Concatenate  Mode=Multidimensional array
  Matrix Concatenation2 : Concatenate  Mode=Multidimensional array  ConcatenateDimension=2
  Matrix Multiply{1..4} (4 alike) : Product  Multiplication=Matrix(*)
  Selector1 : Selector  InputPortWidth=6  IndexOptions=Index vector (dialog)  Indices=[1 2 3]  OutputSizes=1
  Selector2 : Selector  InputPortWidth=6  IndexOptions=Index vector (dialog)  Indices=[4 5 6]  OutputSizes=1
  Skew Symmetrical Operator : Subsystem
  "Skew Symmetrical Operator " : Subsystem
  Submatrix : matrix_library/Submatrix  RowSpan=Range of rows  RowStartMode=Index  RowStartIndex=1  RowEndMode=Index  RowEndIndex=3  ColSpan=Range of columns  ColStartMode=Index  ColStartIndex=1  ColEndMode=Index  ColEndIndex=3
  Submatrix1 : matrix_library/Submatrix  RowSpan=Range of rows  RowStartMode=Index  RowStartIndex=1  RowEndMode=Index  RowEndIndex=3  ColSpan=Range of columns  ColStartMode=Index  ColStartIndex=4  ColEndMode=Index  ColEndIndex=6
  Submatrix2 : matrix_library/Submatrix  RowSpan=Range of rows  RowStartMode=Index  RowStartIndex=4  RowEndMode=Index  RowEndIndex=6  ColSpan=Range of columns  ColStartMode=Index  ColStartIndex=1  ColEndMode=Index  ColEndIndex=3
  Submatrix3 : matrix_library/Submatrix  RowSpan=Range of rows  RowStartMode=Index  RowStartIndex=4  RowEndMode=Index  RowEndIndex=6  ColSpan=Range of columns  ColStartMode=Index  ColStartIndex=4  ColEndMode=Index  ColEndIndex=6
  Subsystem : Subsystem
  Sum2 : Sum  Inputs=|++  SaturateOnIntegerOverflow=on
  Sum3 : Sum  Inputs=|++  SaturateOnIntegerOverflow=on
  Zero matrix (3 x 3) : Constant  Value=zeros(3,3)
  CA_T : Outport  VectorParamsAs1DForOutWhenUnconnected=off
  wires:
  Matrix Concatenation2/1 -> CA_T/1
  nu_T/1 -> Selector1/1, Selector2/1
  Gain2/1 -> Matrix Concatenation1/2  "CA(2,2)"
  Gain1/1 -> Matrix Concatenation/2, Matrix Concatenation1/1  "CA(1,2)"
  Skew Symmetrical Operator/1(S(V)) -> Gain2/1
  "Skew Symmetrical Operator "/1(S(V)) -> Gain1/1
  Sum3/1 -> Skew Symmetrical Operator/1(v)
  Sum2/1 -> "Skew Symmetrical Operator "/1(v)
  Selector2/1 -> Matrix Multiply4/2, Matrix Multiply1/2  "nu_T2"
  Matrix Multiply4/1 -> Sum3/2  "M22 * nu_T2"
  Selector1/1 -> Matrix Multiply3/2, Matrix Multiply2/2  "nu_T1"
  Matrix Multiply3/1 -> Sum3/1  "M21 * nu_T1"
  Matrix Multiply1/1 -> Sum2/2  "M12 * nu_T2"
  Matrix Multiply2/1 -> Sum2/1  "M11 * nu_T1"
  Matrix Concatenation1/1 -> Matrix Concatenation2/2
  Matrix Concatenation/1 -> Matrix Concatenation2/1
  Zero matrix (3 x 3)/1 -> Matrix Concatenation/1  "CA(1,1)"
  Subsystem/1(MA_T) -> Submatrix/1, Submatrix1/1, Submatrix3/1, Submatrix2/1
  Submatrix2/1 -> Matrix Multiply3/1  "M21_T"
  Submatrix3/1 -> Matrix Multiply4/1  "M22_T"
  Submatrix1/1 -> Matrix Multiply1/1  "M12_T"
  Submatrix/1 -> Matrix Multiply2/1  "M11_T"

== system MJAUV_Maneuverability_model_V2/MJ-AUV Model & PropulsionSystem/Dynamics and Kinematics/Subsystem7/Damping forces1 ==
  nu_T : Inport
  Abs : Abs
  Create Diagonal Matrix : matrix_library/Create Diagonal Matrix
  Gain : Gain  Gain=-1
  Linear Damping Matrix : Constant  Value=DL
  Matrix Multiply : Product  Multiplication=Matrix(*)
  Product : Product  SaturateOnIntegerOverflow=on  OutDataTypeStr=Inherit: Same as first input
  Quadratic Damping Vector : Constant  Value=dQ_T
  Reshape1 : Reshape  OutputDimensionality=Column vector (2-D)
  Reshape2 : Reshape  OutputDimensionality=Column vector (2-D)  OutputDimensions=[6,6]
  Sum1 : Sum  Inputs=|++  SaturateOnIntegerOverflow=on
  D * nu_T : Outport  VectorParamsAs1DForOutWhenUnconnected=off
  wires:
  Gain/1 -> Matrix Multiply/1
  Sum1/1 -> Gain/1  "D"
  Matrix Multiply/1 -> D * nu_T/1
  Quadratic Damping Vector/1 -> Reshape2/1  "dQ"
  Abs/1 -> Product/2  "abs(nu_T)"
  Product/1 -> Create Diagonal Matrix/1
  Create Diagonal Matrix/1 -> Sum1/2
  Linear Damping Matrix/1 -> Sum1/1
  nu_T/1 -> Reshape1/1
  Reshape1/1 -> Abs/1, Matrix Multiply/2
  Reshape2/1 -> Product/1

== system MJAUV_Maneuverability_model_V2/MJ-AUV Model & PropulsionSystem/Dynamics and Kinematics/Subsystem7/Restoring forces1 ==
  eta_E : Inport
  B_T : Inport  Port=2
  3x3 Cross Product : sharedutil/3x3 Cross Product  aMode=aMode
  3x3 Cross Product1 : sharedutil/3x3 Cross Product  aMode=aMode
  Constant : Constant  Value=0
  E1(e) : Subsystem
  Gain : Gain  Gain=-1  SaturateOnIntegerOverflow=on  OutDataTypeStr=Inherit: Same as input  ParamDataTypeStr=Inherit: Same as input
  Gain1 : Gain  Gain=-1
  Matrix Multiply : Product  Multiplication=Matrix(*)
  Matrix Multiply1 : Product  Multiplication=Matrix(*)
  Mux : Mux  Inputs=2
  Mux1 : Mux  Inputs=3
  Selector : Selector  InputPortWidth=7  IndexOptions=Index vector (dialog)  Indices=[4 5 6 7]  OutputSizes=1
  Sum1 : Sum  Inputs=|++  SaturateOnIntegerOverflow=on
  Sum2 : Sum  Inputs=|++  SaturateOnIntegerOverflow=on
  Transpose : Math  Operator=transpose  SignedPower=on
  fGT_E : Constant  Value=[0;0;W_T]
  rB_T : Constant  Value=rB_T
  rG_T : Constant  Value=rG_T
  g(eta_E)_T : Outport  VectorParamsAs1DForOutWhenUnconnected=off
  wires:
  eta_E/1 -> Selector/1  "E1(e)"
  Selector/1 -> E1(e)/1(e)  "e"
  Gain/1 -> g(eta_E)_T/1
  Mux/1 -> Gain/1
  Sum2/1 -> Mux/2
  rB_T/1 -> 3x3 Cross Product1/1
  3x3 Cross Product1/1 -> Sum2/2  "rB_T x fG_T"
  3x3 Cross Product/1 -> Sum2/1  "rG_T x fG_T"
  Sum1/1 -> Mux/1  "fG_T + fB_T"
  rG_T/1 -> 3x3 Cross Product/1
  Matrix Multiply1/1 -> 3x3 Cross Product1/2, Sum1/2  "fB_T"
  Matrix Multiply/1 -> 3x3 Cross Product/2, Sum1/1  "fG_T"
  Mux1/1 -> Matrix Multiply1/2  "fBT_E"
  fGT_E/1 -> Matrix Multiply/2
  Transpose/1 -> Matrix Multiply1/1, Matrix Multiply/1  "E1(e)^T"
  E1(e)/1(E1) -> Transpose/1  "E1(e)"
  Constant/1 -> Mux1/2, Mux1/1
  Gain1/1 -> Mux1/3
  B_T/1 -> Gain1/1

== system MJAUV_Maneuverability_model_V2/MJ-AUV Model & PropulsionSystem/Dynamics and Kinematics/Subsystem7/Rigid-body Coriolis and centripetal matrix1 ==
  nu_T : Inport
  Gain : Gain  Gain=mT  SaturateOnIntegerOverflow=on  OutDataTypeStr=Inherit: Same as input  ParamDataTypeStr=Inherit: Same as input
  Gain1 : Gain  Gain=-mT  SaturateOnIntegerOverflow=on  OutDataTypeStr=Inherit: Same as input  ParamDataTypeStr=Inherit: Same as input
  Gain2 : Gain  Gain=-1  SaturateOnIntegerOverflow=on  OutDataTypeStr=Inherit: Same as input  ParamDataTypeStr=Inherit: Same as input
  Matrix Concatenation : Concatenate  Mode=Multidimensional array
  Matrix Concatenation1 : Concatenate  Mode=Multidimensional array
  Matrix Concatenation2 : Concatenate  Mode=Multidimensional array  ConcatenateDimension=2
  Matrix Multiply : Product  Multiplication=Matrix(*)
  Matrix Multiply1 : Product  Multiplication=Matrix(*)
  Matrix Multiply2 : Product  Multiplication=Matrix(*)
  Selector : Selector  InputPortWidth=6  IndexOptions=Index vector (dialog)  Indices=[4 5 6]  OutputSizes=1
  Selector1 : Selector  InputPortWidth=6  IndexOptions=Index vector (dialog)  Indices=[1 2 3]  OutputSizes=1
  "Skew Symmetrical Operator " : Subsystem
  Skew Symmetrical Operator : Subsystem
  "Skew Symmetrical Operator " : Subsystem
  "Skew Symmetrical Operator  " : Subsystem
  Subsystem : Subsystem
  Sum1 : Sum  Inputs=|++  SaturateOnIntegerOverflow=on
  Sum2 : Sum  Inputs=|-+  SaturateOnIntegerOverflow=on
  Zero matrix (3 x 3) : Constant  Value=zeros(3,3)
  rG_T : Constant  Value=rG_T
  CRB_T : Outport  VectorParamsAs1DForOutWhenUnconnected=off
  wires:
  "Skew Symmetrical Operator  "/1(S(V)) -> Matrix Multiply1/2, Matrix Multiply/1  "S(rG_T)"
  Matrix Multiply1/1 -> Sum1/2  "S(nu_T2) * S(rG_T)"
  Sum1/1 -> Gain1/1
  "Skew Symmetrical Operator "/1(S(V)) -> Matrix Multiply1/1, Matrix Multiply/2  "S(nu_T2)"
  Matrix Concatenation/1 -> Matrix Concatenation2/1
  Subsystem/1(Ib_T) -> Matrix Multiply2/1
  Matrix Multiply/1 -> Sum2/2  "S(rG_T) * S(nu_T2)"
  Selector/1 -> Matrix Multiply2/2, "Skew Symmetrical Operator "/1(v)  "nu_T2"
  Matrix Concatenation1/1 -> Matrix Concatenation2/2
  Sum2/1 -> Gain/1
  Matrix Multiply2/1 -> "Skew Symmetrical Operator "/1(v)  "IO * nu_T2"
  Zero matrix (3 x 3)/1 -> Matrix Concatenation/1  "CRB(1,1)"
  Gain1/1 -> Matrix Concatenation1/1  "CRB(1,2)"
  Skew Symmetrical Operator/1(S(V)) -> Sum1/1, Sum2/1  "S(nu_T1)"
  Matrix Concatenation2/1 -> CRB_T/1
  nu_T/1 -> Selector/1, Selector1/1
  Selector1/1 -> Skew Symmetrical Operator/1(v)  "nu_T1"
  "Skew Symmetrical Operator "/1(S(V)) -> Gain2/1  "S(IO * nu_T2)"
  rG_T/1 -> "Skew Symmetrical Operator  "/1(v), Subsystem/1(rG_T)  "rG_T"
  Gain/1 -> Matrix Concatenation/2  "CRB(2,1)"
  Gain2/1 -> Matrix Concatenation1/2  "CRB(2,2)"

== system MJAUV_Maneuverability_model_V2/MJ-AUV Model & PropulsionSystem/Dynamics and Kinematics/Subsystem7/Subsystem1 ==
  eta_E_B : Inport
  Theta : Inport  Port=2
  Demux : Demux  Outputs=3
  Mux : Mux  Inputs=3
  Mux1 : Mux  Inputs=2
  Quaternion normalisation : Subsystem
  Quaternions to Euler Angles : Subsystem
  Selector : Selector  InputPortWidth=7  IndexOptions=Index vector (dialog)  Indices=[4 5 6 7]  OutputSizes=1
  Selector1 : Selector  InputPortWidth=3  IndexOptions=Index vector (dialog)  Indices=[1]  OutputSizes=1
  Selector2 : Selector  InputPortWidth=7  IndexOptions=Index vector (dialog)  Indices=[1 2 3]  OutputSizes=1
  Selector3 : Selector  InputPortWidth=3  IndexOptions=Index vector (dialog)  Indices=[2]  OutputSizes=1
  Subsystem : Subsystem
  Subsystem1 : Subsystem
  Sum : Sum  Inputs=||+++
  eta_E_T : Outport
  wires:
  eta_E_B/1 -> Selector2/1, Selector/1
  Selector/1 -> Quaternions to Euler Angles/1(Quaternions)  "e"
  Demux/2 -> Mux/2
  Demux/3 -> Sum/1
  Quaternions to Euler Angles/1(Euler Angles) -> Demux/1
  Subsystem/1(Quaternions) -> Mux1/2
  Selector1/1 -> Sum/2  "Theta1"
  Selector2/1 -> Mux1/1  "e"
  Mux/1 -> Subsystem/1("Euler Angles ")
  Demux/1 -> Mux/1
  Mux1/1 -> Quaternion normalisation/1(eta_E)
  Sum/1 -> Subsystem1/1(In2)
  Quaternion normalisation/1(eta_E (norm)) -> eta_E_T/1
  Theta/1 -> Selector3/1, Selector1/1
  Selector3/1 -> Sum/3  "Theta2"
  Subsystem1/1(Out1) -> Mux/3

== system MJAUV_Maneuverability_model_V2/MJ-AUV Model & PropulsionSystem/Dynamics and Kinematics/Subsystem8/Added Mass Coriolis and centripetal matrix1 ==
  nu_F : Inport
  Gain1 : Gain  Gain=-1  SaturateOnIntegerOverflow=on  OutDataTypeStr=Inherit: Same as input  ParamDataTypeStr=Inherit: Same as input
  Gain2 : Gain  Gain=-1  SaturateOnIntegerOverflow=on  OutDataTypeStr=Inherit: Same as input  ParamDataTypeStr=Inherit: Same as input
  Matrix Concatenation : Concatenate  Mode=Multidimensional array
  Matrix Concatenation1 : Concatenate  Mode=Multidimensional array
  Matrix Concatenation2 : Concatenate  Mode=Multidimensional array  ConcatenateDimension=2
  Matrix Multiply{1..4} (4 alike) : Product  Multiplication=Matrix(*)
  Selector1 : Selector  InputPortWidth=6  IndexOptions=Index vector (dialog)  Indices=[1 2 3]  OutputSizes=1
  Selector2 : Selector  InputPortWidth=6  IndexOptions=Index vector (dialog)  Indices=[4 5 6]  OutputSizes=1
  Skew Symmetrical Operator : Subsystem
  "Skew Symmetrical Operator " : Subsystem
  Submatrix : matrix_library/Submatrix  RowSpan=Range of rows  RowStartMode=Index  RowStartIndex=1  RowEndMode=Index  RowEndIndex=3  ColSpan=Range of columns  ColStartMode=Index  ColStartIndex=1  ColEndMode=Index  ColEndIndex=3
  Submatrix1 : matrix_library/Submatrix  RowSpan=Range of rows  RowStartMode=Index  RowStartIndex=1  RowEndMode=Index  RowEndIndex=3  ColSpan=Range of columns  ColStartMode=Index  ColStartIndex=4  ColEndMode=Index  ColEndIndex=6
  Submatrix2 : matrix_library/Submatrix  RowSpan=Range of rows  RowStartMode=Index  RowStartIndex=4  RowEndMode=Index  RowEndIndex=6  ColSpan=Range of columns  ColStartMode=Index  ColStartIndex=1  ColEndMode=Index  ColEndIndex=3
  Submatrix3 : matrix_library/Submatrix  RowSpan=Range of rows  RowStartMode=Index  RowStartIndex=4  RowEndMode=Index  RowEndIndex=6  ColSpan=Range of columns  ColStartMode=Index  ColStartIndex=4  ColEndMode=Index  ColEndIndex=6
  Subsystem : Subsystem
  Sum2 : Sum  Inputs=|++  SaturateOnIntegerOverflow=on
  Sum3 : Sum  Inputs=|++  SaturateOnIntegerOverflow=on
  Zero matrix (3 x 3) : Constant  Value=zeros(3,3)
  CA_F : Outport  VectorParamsAs1DForOutWhenUnconnected=off
  wires:
  Zero matrix (3 x 3)/1 -> Matrix Concatenation/1  "CA(1,1)"
  Matrix Concatenation/1 -> Matrix Concatenation2/1
  Matrix Concatenation1/1 -> Matrix Concatenation2/2
  Matrix Multiply2/1 -> Sum2/1  "M11 * nu_F1"
  Matrix Multiply1/1 -> Sum2/2  "M12 * nu_F2"
  Matrix Multiply3/1 -> Sum3/1  "M21 * nu_F1"
  Selector1/1 -> Matrix Multiply2/2, Matrix Multiply3/2  "nu_F1"
  Matrix Multiply4/1 -> Sum3/2  "M22 * nu_F2"
  Selector2/1 -> Matrix Multiply1/2, Matrix Multiply4/2  "nu_F2"
  Sum2/1 -> "Skew Symmetrical Operator "/1(v)
  Sum3/1 -> Skew Symmetrical Operator/1(v)
  "Skew Symmetrical Operator "/1(S(V)) -> Gain1/1
  Skew Symmetrical Operator/1(S(V)) -> Gain2/1
  Gain1/1 -> Matrix Concatenation1/1, Matrix Concatenation/2  "CA(1,2)"
  Gain2/1 -> Matrix Concatenation1/2  "CA(2,2)"
  nu_F/1 -> Selector2/1, Selector1/1
  Matrix Concatenation2/1 -> CA_F/1
  Subsystem/1(MA_F) -> Submatrix3/1, Submatrix2/1, Submatrix/1, Submatrix1/1
  Submatrix2/1 -> Matrix Multiply3/1  "M21_F"
  Submatrix3/1 -> Matrix Multiply4/1  "M22_F"
  Submatrix1/1 -> Matrix Multiply1/1  "M12_F"
  Submatrix/1 -> Matrix Multiply2/1  "M11_F"
